simulink model "space-state"  (R2014b)
settings: Solver=ode14x  StartTime=0.0  StopTime=inf  FixedStep=0.1  RelTol=1e-3
undefined symbols (not defined in the file or in its folder): A, B, C, K, L
libraries: arduino_io_lib x1
settings Model: Creator=mtsou_000  LastModifiedBy=mtsou_000

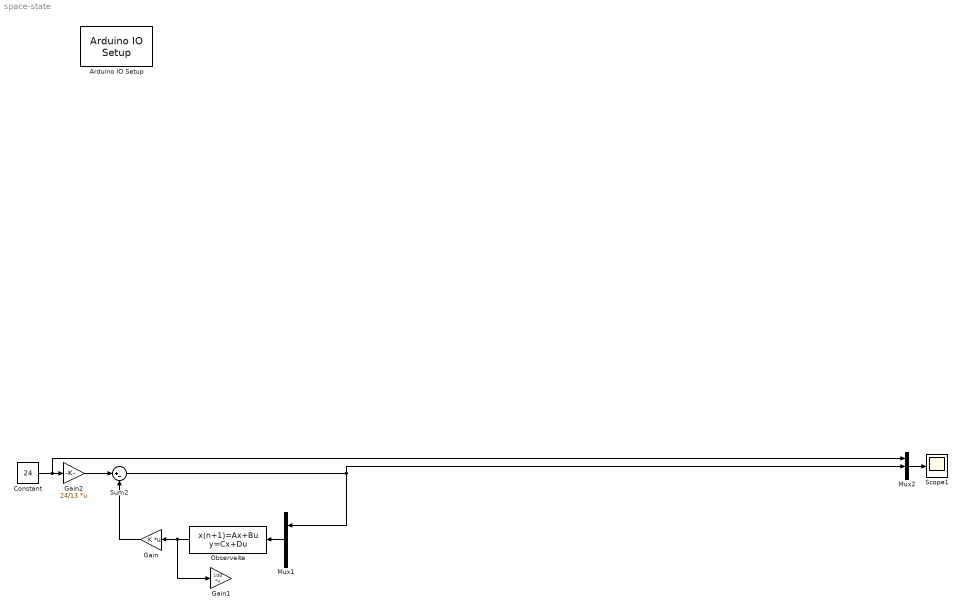
== system space-state ==
  Arduino IO Setup : arduino_io_lib/Arduino IO Setup  Priority=3  arduinoVar=Temporary arduino variable: Arduino1  workspaceVarName=a  comPort=COM8
  Constant : Constant  Value=24
  Gain : Gain  Gain=K  Multiplication=Matrix(K*u)
  Gain1 : Gain  Gain=100  Multiplication=Matrix(K*u)
  Gain2 : Gain  Gain=24/13  Multiplication=Matrix(K*u)
  Mux1 : Mux  Inputs=2
  Mux2 : Mux  Inputs=3
  Observeite : DiscreteStateSpace  A=A-L*C  B=[B L]  C=eye(2)  D=zeros(2)  SampleTime=0.1
  Scope1 : Scope
      settings: TimeRange=10  YMin=0  YMax=35  SaveName=ScopeData3
  Sum2 : Sum  Inputs=|+-
  wires:
  Observeite/1 -> Gain1/1, Gain/1
  Mux1/1 -> Observeite/1
  Mux2/1 -> Scope1/1
  Gain/1 -> Sum2/2
  Constant/1 -> Mux2/1, Gain2/1
  Sum2/1 -> Mux1/1, Mux2/2
  Gain2/1 -> Sum2/1
